simulink model "matlabfcn"  (R2021a)
settings: Solver=FixedStepDiscrete  StartTime=0.0  StopTime=10.0  RelTol=1e-3
CloseFcn:
  | clear all
  | try
  | rmdir slprj\ s
  | catch
  | end
  | try
  | folder_name = [bdroot '*'];
  | rmdir(folder_name,'s')
  | catch
  | end
  | try
  | file_temp_name = [bdroot '.slxc'];
  | delete(file_temp_name)
  | delete *.mexw64
  | catch
  | end
  | clear folder_name file_temp_name
settings Model: Creator=jetson  LastModifiedBy=jetson
settings DataIOCC: SaveOutput=off  SignalLogging=off  DSMLogging=off  SaveTime=off  ReturnWorkspaceOutputs=off
settings OptimizationCC: DefaultParameterBehavior=Inlined  EnhancedBackFolding=on  PassReuseOutputArgsAs=Individual arguments  ZeroExternalMemoryAtStartup=off  ZeroInternalMemoryAtStartup=off  OptimizeBlockOrder=speed  DifferentSizesBufferReuse=on  OptimizationCustomize=off  EfficientTunableParamExpr=on
settings DebuggingCC: ParameterTunabilityLossMsg=error
settings SFSimCC: SimCustomHeaderCode="#include \"doubleIt.h\""  SimUserSources=doubleIt.c  MATLABDynamicMemAlloc=off
settings RTWCC: SystemTargetFile=ert.tlc  GenCodeOnly=on  TemplateMakefile=ert_default_tmf  GenerateReport=on  RTWUseSimCustomCode=on  CustomHeaderCode="#include \"doubleIt.h\""  CustomSource=doubleIt.c  IncludeHyperlinkInReport=on  LaunchReport=on  GenerateTraceInfo=on
settings CodeAppCC: ForceParamTrailComments=on  IgnoreCustomStorageClasses=off  OperatorAnnotations=on  SimulinkDataObjDesc=on  SFDataObjDesc=on  InsertBlockDesc=on
settings ERTTargetCC: TargetLangStandard=C99 (ISO)  GenerateSampleERTMain=on  InlinedParameterPlacement=NonHierarchical  ERTCustomFileTemplate=example_file_process.tlc

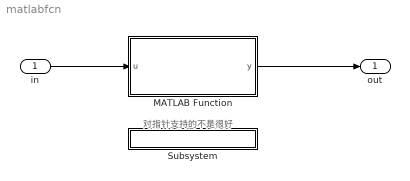
== system matlabfcn ==
  note: 对指针支持的不是很好
  in : Inport  ClipboardFcn=Data Type : %<OutDataTypeStr>  OutDataTypeStr=double
      settings: AttributesFormatString=Data Type : %<OutDataTypeStr>
  MATLAB Function : MATLAB Function  TreatAsAtomicUnit=on
  Subsystem : Subsystem
      settings: OpenFcn=web(fullfile(docroot, 'simulink/ug/incorporate-c-code-using-a-matlab-function-block.html'))
      mask Display: disp('double click open help')
  out : Outport  OutDataTypeStr=double
      settings: AttributesFormatString=Data Type : %<OutDataTypeStr>
  wires:
  in/1 -> MATLAB Function/1(u)
  MATLAB Function/1(y) -> out/1

== system matlabfcn/Subsystem ==

== matlab function matlabfcn/MATLAB Function ==
  data: u input; y output
function y = callingDoubleIt(u)

y = 0.0;
y = coder.ceval('doubleIt',u);
